simulink model "edsonSimulation"  (R2025b)
settings: Solver=ode4  StartTime=0.0  StopTime=100  FixedStep=1e-3  RelTol=1e-3
values from neighbouring files (symbols this model uses):
  c1 = input(40)    [control_ABFTISMC.m]
  D = [13.9269190731477, 0.478984747386228, 13.9043475853434, 0.479066331803849 ... (first row only)    [Hinf.m]    (also in control_ABFTISMC.m = [input(19), input(20), input(21); dinamic.m = - [X_u + X_uu * abs(u),              0,                   0; linealization.m = - [coef.X_u + coef.X_uu * abs(u_sym),              0,       )
  gamma = [atan2(diff(y_smooth),diff(x_smooth)), atan2(diff(y_smooth(end-1:end)),diff(x_smooth(end-1:end)))]    [trajectory.m]
  h1 = input(50)    [control_ABFTISMC.m]
  h2 = input(51)    [control_ABFTISMC.m]
  h3 = input(53)    [control_ABFTISMC.m]
  I_z = input(12)    [dinamic.m]    (also in linealization.m = coef.I_z; simulationParameters.m = 204.1)
  lambda1 = input(57)    [control_ABFTISMC.m]
  lambda2 = input(52)    [control_ABFTISMC.m]
  M = [input(1), input(2), input(3) ... (first row only)    [control_ABFTISMC.m]    (also in dinamic.m = [m - X_u_dot,           0,                      0; hinfController.m = 1.5; linealization.m = [coef.m - X_u_dot,           0,                      0)
  m = input(6)    [dinamic.m]    (also in simulationParameters.m = 250)
  N_ncnd = input(29)    [dinamic.m]    (also in simulationParameters.m = -1.5777)
  N_r = input(18)    [dinamic.m]    (also in simulationParameters.m = -741.1947; trajectory_2.m = 8.68555609659)
  N_r_dot = input(13)    [dinamic.m]    (also in linealization.m = coef.N_r_dot; simulationParameters.m = -748.3102)
  N_rnc = input(27)    [dinamic.m]    (also in simulationParameters.m = -2.8549)
  N_rr = input(19)    [dinamic.m]    (also in simulationParameters.m = -262.7909)
  N_und = input(28)    [dinamic.m]    (also in simulationParameters.m = 2.7616)
  N_v_dot = input(11)    [dinamic.m]    (also in linealization.m = coef.N_v_dot; simulationParameters.m = -370.5973)
  N_vnc = input(26)    [dinamic.m]    (also in simulationParameters.m = -0.5382)
  p = input(47)    [control_ABFTISMC.m]
  phi1 = input(49)    [control_ABFTISMC.m]
  q = input(48)    [control_ABFTISMC.m]
  r_0 = eps    [linealization.m]    (also in simulationParameters.m = 0)
  u_0 = 2.0    (= 2)    [linealization.m]    (also in simulationParameters.m = 0)
  v_0 = eps    [linealization.m]    (also in simulationParameters.m = 0)
  x_0 = 0    [linealization.m]    (also in simulationParameters.m)
  x_g = input(10)    [dinamic.m]    (also in linealization.m = coef.x_g; simulationParameters.m = 0.08)
  X_ncnc = input(22)    [dinamic.m]    (also in simulationParameters.m = 1.0518)
  X_ndnd = input(23)    [dinamic.m]    (also in simulationParameters.m = 1.0518)
  X_rnd = input(21)    [dinamic.m]    (also in simulationParameters.m = 1.8411)
  X_u = input(14)    [dinamic.m]    (also in simulationParameters.m = -0.2912)
  X_u_dot = input(7)    [dinamic.m]    (also in linealization.m = coef.X_u_dot; simulationParameters.m = -2.4706)
  X_unc = input(20)    [dinamic.m]    (also in simulationParameters.m = -3.6822)
  X_uu = input(15)    [dinamic.m]    (also in simulationParameters.m = -27.6262)
  y_0 = 0    [linealization.m]    (also in simulationParameters.m)
  Y_r_dot = input(9)    [dinamic.m]    (also in linealization.m = coef.Y_r_dot; simulationParameters.m = -370.5973)
  Y_rnc = -0.5382    [simulationParameters.m]
  Y_v = input(16)    [dinamic.m]    (also in simulationParameters.m = -123.5324)
  Y_v_dot = input(8)    [dinamic.m]    (also in linealization.m = coef.Y_v_dot; simulationParameters.m = -247.0649)
  Y_vnc = input(24)    [dinamic.m]    (also in simulationParameters.m = -0.3588)
  Y_vv = input(17)    [dinamic.m]    (also in simulationParameters.m = -38.9275)
  yaw_0 = 0    [linealization.m]    (also in simulationParameters.m)
undefined symbols (not defined in the file or in its folder): mu, set_point
settings Model: Creator=b_ant  LastModifiedBy=b_ant

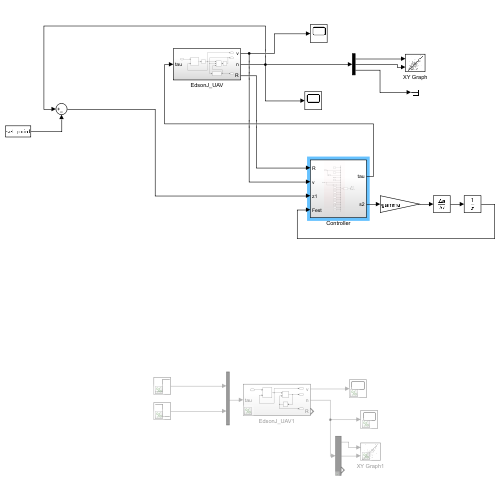
[thumbnail: Simulink's stored preview of the top-level diagram]
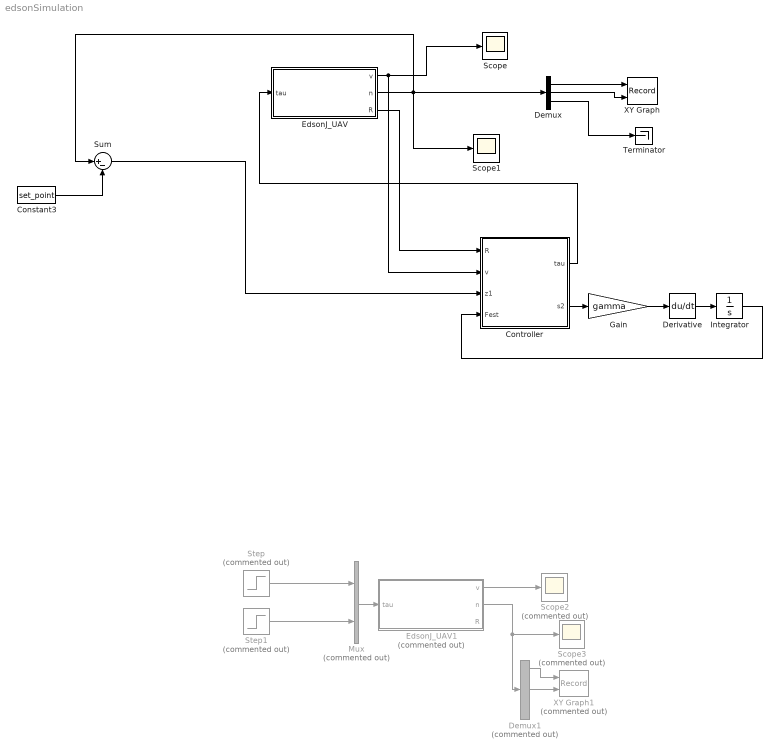
== system edsonSimulation ==
  Constant3 : Constant  Value=set_point
  Controller : Subsystem
  Demux : Demux  Outputs=3
  Demux1 : Demux  Commented=on  Outputs=3
  Derivative : Derivative
  EdsonJ_UAV : Subsystem
  EdsonJ_UAV1 : Subsystem  Commented=on
  Gain : Gain  Gain=gamma
  Integrator : Integrator  InitialCondition=[0,0,0]'
  Mux : Mux  Commented=on  Inputs=2
  Scope : Scope
      settings: ActiveDisplayYMinimum=-2.1186471793877021E+26  ActiveDisplayYMaximum=4.478113109634338E+26
  Scope1 : Scope
      settings: ActiveDisplayYMinimum=-3.5145777569055263E+26  ActiveDisplayYMaximum=4.6906781291110869E+26
  Scope2 : Scope  Commented=on
      settings: ActiveDisplayYMinimum=-0.014674055128684147  ActiveDisplayYMaximum=0.13206649615815735  DataLoggingVariableName=ScopeData2
  Scope3 : Scope  Commented=on
      settings: ActiveDisplayYMinimum=-2.3702438288098757  ActiveDisplayYMaximum=21.081039558840153  DataLoggingVariableName=ScopeData3
  Step : Step  Commented=on  After=0  SampleTime=0
  Step1 : Step  Commented=on  Before=100  After=0  SampleTime=0
  Sum : Sum  Inputs=|+-
  Terminator : Terminator
  XY Graph : Record  NumPorts=2.0  FileSettingsInternal="{\"entries\":[{\"content\":{\"excelSettings\":{\"content\":{},\"type\":\"Streamout.ExcelSettings\"},\"parquetSettings\":{\"content\":{},\"type\":\"Streamout.ParquetSettings\"}},\"type\":\"Streamout.FileSettingStorage\",\"uuid\":\"\"}],\"packageUris\":[\"http:\\/\\/schema.mathworks.com\\/mf0\\/streamout_blocks\\/R2020a\"],\"version\":\"1.0\"}"  FrameSettings=[0, 0]  Layout=[1 1]  SignalsInternal="{\"entries\":[{\"content\":{\"signals\":[{\"content\":{\"blockPath\":[],\"dimensions\":[1],\"domain\":\"\",\"lineColor\":\"#a2142f\",\"plots\":[ 1 ],\"port\":1,\"signalID\":1,\"signalName\":\"Demux:1\"},\"type\":\"RecordBlkView.Signal\",\"uuid\":\"\"},{\"content\":{\"blockPath\":[],\"dimensions\":[1],\"domain\":\"\",\"lineColor\":\"#139fff\",\"plots\":[ 1 ],\"port\":2,\"signalID\":2,\"signalName\":\"Demux:2\"},\"type\":\"RecordBlkView.Signal\",\"uuid\":\"\"}]},\"type\":\"RecordBlkView.InputSignals\",\"uuid\":\"\"}],\"packageUris\":[\"http:\\/\\/schema.mathworks.com\\/mf0\\/streamout_blocks\\/R2020a\"],\"version\":\"1.0\"}"  VisualizationBindings="{\"xyplotplugin\":{\"info\":[{\"series\":[{\"bindingParametersList\":[{\"parameter\":\"X-Axis\",\"signalID\":1,\"signalName\":\"Demux:1\"},{\"parameter\":\"Y-Axis\",\"signalID\":2,\"signalName\":\"Demux:2\"}],\"seriesID\":0}],\"subplotID\":1}]}}"  CompatibilityTag=XY
  XY Graph1 : Record  Commented=on  NumPorts=2.0  FileSettingsInternal="{\"entries\":[{\"content\":{\"excelSettings\":{\"content\":{},\"type\":\"Streamout.ExcelSettings\"},\"parquetSettings\":{\"content\":{},\"type\":\"Streamout.ParquetSettings\"}},\"type\":\"Streamout.FileSettingStorage\",\"uuid\":\"\"}],\"packageUris\":[\"http:\\/\\/schema.mathworks.com\\/mf0\\/streamout_blocks\\/R2020a\"],\"version\":\"1.0\"}"  FrameSettings=[0, 0]  Layout=[1 1]  SignalsInternal="{\"entries\":[{\"content\":{\"signals\":[{\"content\":{\"blockPath\":[],\"dimensions\":[1],\"domain\":\"\",\"lineColor\":\"#a2142f\",\"plots\":[ 1 ],\"port\":1,\"signalID\":1,\"signalName\":\"Demux1:1\"},\"type\":\"RecordBlkView.Signal\",\"uuid\":\"\"},{\"content\":{\"blockPath\":[],\"dimensions\":[1],\"domain\":\"\",\"lineColor\":\"#139fff\",\"plots\":[ 1 ],\"port\":2,\"signalID\":2,\"signalName\":\"Demux1:2\"},\"type\":\"RecordBlkView.Signal\",\"uuid\":\"\"}]},\"type\":\"RecordBlkView.InputSignals\",\"uuid\":\"\"}],\"packageUris\":[\"http:\\/\\/schema.mathworks.com\\/mf0\\/streamout_blocks\\/R2020a\"],\"version\":\"1.0\"}"  VisualizationBindings="{\"xyplotplugin\":{\"info\":[{\"series\":[{\"bindingParametersList\":[{\"parameter\":\"X-Axis\",\"signalID\":1,\"signalName\":\"Demux1:1\"},{\"parameter\":\"Y-Axis\",\"signalID\":2,\"signalName\":\"Demux1:2\"}],\"seriesID\":0}],\"subplotID\":1}]}}"  CompatibilityTag=XY
  wires:
  EdsonJ_UAV/1(v) -> Scope/1, Controller/2(v)
  Demux/1 -> XY Graph/1
  Demux/2 -> XY Graph/2
  EdsonJ_UAV/3(R) -> Controller/1(R)
  Constant3/1 -> Sum/2
  Sum/1 -> Controller/3(z1)
  Controller/1(tau) -> EdsonJ_UAV/1(tau)
  Controller/2(s2) -> Gain/1
  Gain/1 -> Derivative/1
  Derivative/1 -> Integrator/1
  Integrator/1 -> Controller/4(Fest)
  Demux/3 -> Terminator/1
  EdsonJ_UAV/2(n) -> Sum/1, Demux/1, Scope1/1
  Mux/1 -> EdsonJ_UAV1/1(tau)
  Step1/1 -> Mux/2
  Step/1 -> Mux/1
  EdsonJ_UAV1/2(n) -> Demux1/1, Scope3/1
  EdsonJ_UAV1/1(v) -> Scope2/1
  Demux1/2 -> XY Graph1/2
  Demux1/1 -> XY Graph1/1

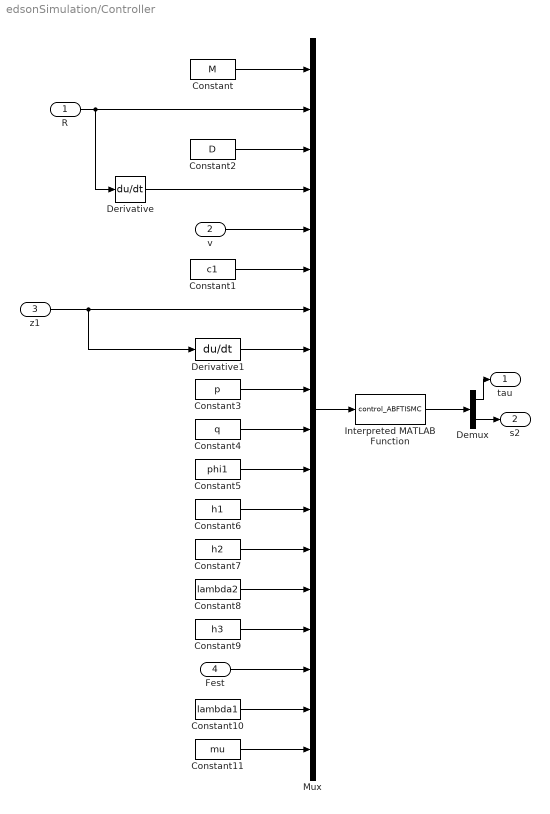
== system edsonSimulation/Controller ==
  R : Inport
  v : Inport  Port=2
  z1 : Inport  Port=3
  Fest : Inport  Port=4
  Constant : Constant  Value=M
  Constant1 : Constant  Value=c1
  Constant10 : Constant  Value=lambda1
  Constant11 : Constant  Value=mu
  Constant2 : Constant  Value=D
  Constant3 : Constant  Value=p
  Constant4 : Constant  Value=q
  Constant5 : Constant  Value=phi1
  Constant6 : Constant  Value=h1
  Constant7 : Constant  Value=h2
  Constant8 : Constant  Value=lambda2
  Constant9 : Constant  Value=h3
  Demux : Demux  Outputs=2
  Derivative : Derivative
  Derivative1 : Derivative
  Interpreted MATLAB Function : MATLABFcn  MATLABFcn=control_ABFTISMC
  Mux : Mux  Inputs=18
  tau : Outport
  s2 : Outport  Port=2
  wires:
  Mux/1 -> Interpreted MATLAB Function/1
  Constant/1 -> Mux/1
  R/1 -> Derivative/1, Mux/2
  Constant2/1 -> Mux/3
  Derivative/1 -> Mux/4
  v/1 -> Mux/5
  Constant1/1 -> Mux/6
  z1/1 -> Derivative1/1, Mux/7
  Derivative1/1 -> Mux/8
  Constant3/1 -> Mux/9
  Constant4/1 -> Mux/10
  Constant5/1 -> Mux/11
  Constant6/1 -> Mux/12
  Constant7/1 -> Mux/13
  Constant8/1 -> Mux/14
  Constant9/1 -> Mux/15
  Fest/1 -> Mux/16
  Interpreted MATLAB Function/1 -> Demux/1
  Demux/2 -> s2/1
  Demux/1 -> tau/1
  Constant10/1 -> Mux/17
  Constant11/1 -> Mux/18

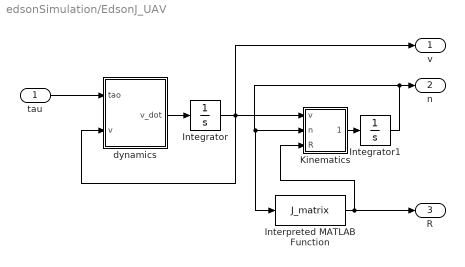
== system edsonSimulation/EdsonJ_UAV ==
  tau : Inport
  Integrator : Integrator  InitialCondition=[0,0,0]
  Integrator1 : Integrator  InitialCondition=[0,0,0]
  Interpreted MATLAB Function : MATLABFcn  MATLABFcn=J_matrix
  Kinematics : Subsystem
  dynamics : Subsystem
  v : Outport
  n : Outport  Port=2
  R : Outport  Port=3
  wires:
  Integrator/1 -> dynamics/2(v), v/1, Kinematics/1(v)
  dynamics/1(v_dot) -> Integrator/1
  Kinematics/1(n_dot) -> Integrator1/1
  Integrator1/1 -> n/1, Interpreted MATLAB Function/1, Kinematics/2(n)
  tau/1 -> dynamics/1(tao)
  Interpreted MATLAB Function/1 -> Kinematics/3(R), R/1

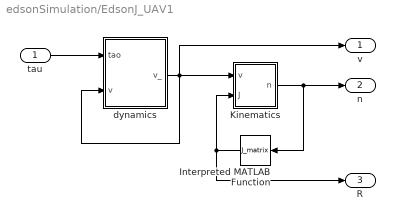
== system edsonSimulation/EdsonJ_UAV1 ==
  tau : Inport
  Interpreted MATLAB Function : MATLABFcn  MATLABFcn=J_matrix
  Kinematics : Subsystem
  dynamics : Subsystem
  v : Outport
  n : Outport  Port=2
  R : Outport  Port=3
  wires:
  dynamics/1(v_) -> Kinematics/1(v), dynamics/2(v), v/1
  Kinematics/1(n) -> n/1, Interpreted MATLAB Function/1
  tau/1 -> dynamics/1(tao)
  Interpreted MATLAB Function/1 -> R/1, Kinematics/2(J)

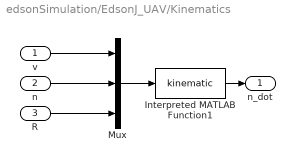
== system edsonSimulation/EdsonJ_UAV/Kinematics ==
  v : Inport
  n : Inport  Port=2
  R : Inport  Port=3
  Interpreted MATLAB Function1 : MATLABFcn  MATLABFcn=kinematic
  Mux : Mux  Inputs=3
  n_dot : Outport
  wires:
  n/1 -> Mux/2
  Mux/1 -> Interpreted MATLAB Function1/1
  v/1 -> Mux/1
  Interpreted MATLAB Function1/1 -> n_dot/1
  R/1 -> Mux/3

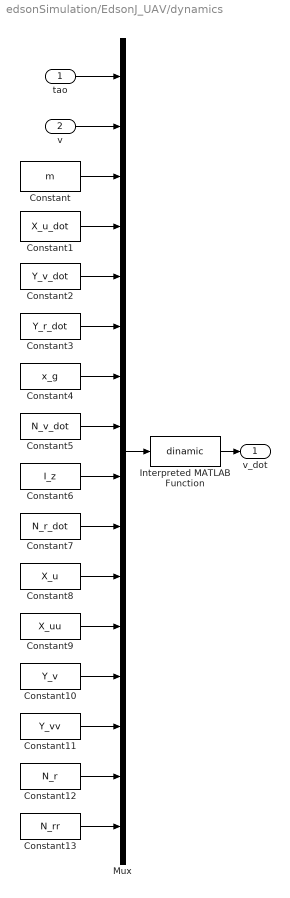
== system edsonSimulation/EdsonJ_UAV/dynamics ==
  tao : Inport
  v : Inport  Port=2
  Constant : Constant  Value=m
  Constant1 : Constant  Value=X_u_dot
  Constant10 : Constant  Value=Y_v
  Constant11 : Constant  Value=Y_vv
  Constant12 : Constant  Value=N_r
  Constant13 : Constant  Value=N_rr
  Constant2 : Constant  Value=Y_v_dot
  Constant3 : Constant  Value=Y_r_dot
  Constant4 : Constant  Value=x_g
  Constant5 : Constant  Value=N_v_dot
  Constant6 : Constant  Value=I_z
  Constant7 : Constant  Value=N_r_dot
  Constant8 : Constant  Value=X_u
  Constant9 : Constant  Value=X_uu
  Interpreted MATLAB Function : MATLABFcn  MATLABFcn=dinamic
  Mux : Mux  Inputs=16
  v_dot : Outport
  wires:
  tao/1 -> Mux/1
  Constant3/1 -> Mux/6
  Constant1/1 -> Mux/4
  Mux/1 -> Interpreted MATLAB Function/1
  v/1 -> Mux/2
  Constant/1 -> Mux/3
  Constant10/1 -> Mux/13
  Constant4/1 -> Mux/7
  Constant13/1 -> Mux/16
  Constant2/1 -> Mux/5
  Constant12/1 -> Mux/15
  Constant9/1 -> Mux/12
  Constant5/1 -> Mux/8
  Constant6/1 -> Mux/9
  Constant11/1 -> Mux/14
  Constant8/1 -> Mux/11
  Constant7/1 -> Mux/10
  Interpreted MATLAB Function/1 -> v_dot/1

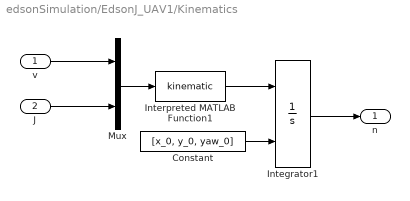
== system edsonSimulation/EdsonJ_UAV1/Kinematics ==
  v : Inport
  J : Inport  Port=2
  Constant : Constant  Value=[x_0, y_0, yaw_0]
  Integrator1 : Integrator  InitialConditionSource=external  InitialCondition=[0,0,0]
  Interpreted MATLAB Function1 : MATLABFcn  MATLABFcn=kinematic
  Mux : Mux  Inputs=2
  n : Outport
  wires:
  Mux/1 -> Interpreted MATLAB Function1/1
  v/1 -> Mux/1
  J/1 -> Mux/2
  Interpreted MATLAB Function1/1 -> Integrator1/1
  Integrator1/1 -> n/1
  Constant/1 -> Integrator1/2

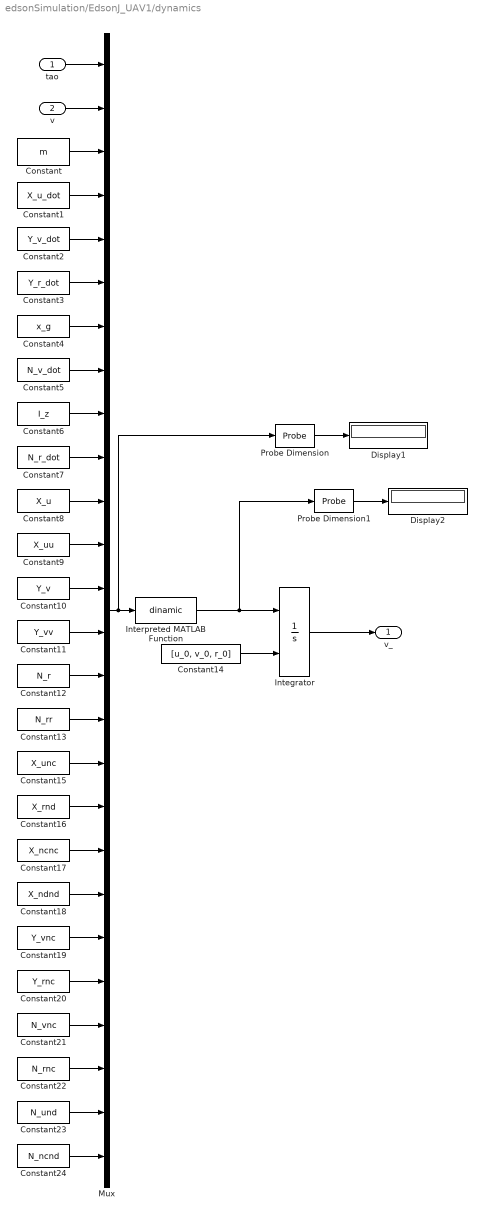
== system edsonSimulation/EdsonJ_UAV1/dynamics ==
  tao : Inport
  v : Inport  Port=2
  Constant : Constant  Value=m
  Constant1 : Constant  Value=X_u_dot
  Constant10 : Constant  Value=Y_v
  Constant11 : Constant  Value=Y_vv
  Constant12 : Constant  Value=N_r
  Constant13 : Constant  Value=N_rr
  Constant14 : Constant  Value=[u_0, v_0, r_0]
  Constant15 : Constant  Value=X_unc
  Constant16 : Constant  Value=X_rnd
  Constant17 : Constant  Value=X_ncnc
  Constant18 : Constant  Value=X_ndnd
  Constant19 : Constant  Value=Y_vnc
  Constant2 : Constant  Value=Y_v_dot
  Constant20 : Constant  Value=Y_rnc
  Constant21 : Constant  Value=N_vnc
  Constant22 : Constant  Value=N_rnc
  Constant23 : Constant  Value=N_und
  Constant24 : Constant  Value=N_ncnd
  Constant3 : Constant  Value=Y_r_dot
  Constant4 : Constant  Value=x_g
  Constant5 : Constant  Value=N_v_dot
  Constant6 : Constant  Value=I_z
  Constant7 : Constant  Value=N_r_dot
  Constant8 : Constant  Value=X_u
  Constant9 : Constant  Value=X_uu
  Display1 : Display
  Display2 : Display
  Integrator : Integrator  InitialConditionSource=external  InitialCondition=[0,0,0]
  Interpreted MATLAB Function : MATLABFcn  MATLABFcn=dinamic
  Mux : Mux  Inputs=26
  Probe Dimension : Probe  ProbeWidth=off  ProbeSampleTime=off  ProbeComplexSignal=off  ProbeSignalDimensions=on
  Probe Dimension1 : Probe  ProbeWidth=off  ProbeSampleTime=off  ProbeComplexSignal=off  ProbeSignalDimensions=on
  v_ : Outport
  wires:
  tao/1 -> Mux/1
  Constant3/1 -> Mux/6
  Constant1/1 -> Mux/4
  Mux/1 -> Probe Dimension/1, Interpreted MATLAB Function/1
  v/1 -> Mux/2
  Constant/1 -> Mux/3
  Constant10/1 -> Mux/13
  Constant4/1 -> Mux/7
  Constant13/1 -> Mux/16
  Constant2/1 -> Mux/5
  Constant12/1 -> Mux/15
  Constant9/1 -> Mux/12
  Constant5/1 -> Mux/8
  Constant6/1 -> Mux/9
  Constant11/1 -> Mux/14
  Constant8/1 -> Mux/11
  Constant7/1 -> Mux/10
  Integrator/1 -> v_/1
  Constant14/1 -> Integrator/2
  Constant15/1 -> Mux/17
  Constant16/1 -> Mux/18
  Constant17/1 -> Mux/19
  Constant18/1 -> Mux/20
  Constant19/1 -> Mux/21
  Constant20/1 -> Mux/22
  Constant21/1 -> Mux/23
  Constant22/1 -> Mux/24
  Constant23/1 -> Mux/25
  Constant24/1 -> Mux/26
  Probe Dimension/1 -> Display1/1
  Interpreted MATLAB Function/1 -> Probe Dimension1/1, Integrator/1
  Probe Dimension1/1 -> Display2/1
